simulink model "rw_assembly_step_ramp_test_rpm_commands"  (R2018b)
settings: Solver=FixedStepAuto  StartTime=0.0  StopTime=200  FixedStep=simParams.sample_time_s  RelTol=1e-3
libraries: simulink x1, reaction_wheel_assembly_lib_disc x1
settings Model: Creator=colem  LastModifiedBy=colem

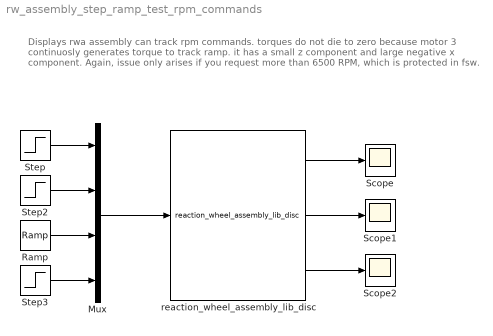
== system rw_assembly_step_ramp_test_rpm_commands ==
  note: Displays rwa assembly can track rpm commands. torques do not die to zero because motor 3 continuosly generates torque to track ramp. it has a small z component and large negative x component. Again, issue only arises if you request more than 6500 RPM, which is protected in fsw.
  Mux : Mux
  Ramp : simulink/Sources/Ramp  slope=6  start=0  InitialOutput=0
  Scope : Scope
  Scope1 : Scope
  Scope2 : Scope
  Step : Step  After=1000  SampleTime=0
  Step2 : Step  After=3000  SampleTime=0
  Step3 : Step  After=-2500  SampleTime=0
  reaction_wheel_assembly_lib_disc : reaction_wheel_assembly_lib_disc/reaction_wheel_assembly_lib_disc  SystemSampleTime=-1
  wires:
  reaction_wheel_assembly_lib_disc/1 -> Scope/1
  reaction_wheel_assembly_lib_disc/2 -> Scope1/1
  reaction_wheel_assembly_lib_disc/3 -> Scope2/1
  Step/1 -> Mux/1
  Step3/1 -> Mux/4
  Step2/1 -> Mux/2
  Mux/1 -> reaction_wheel_assembly_lib_disc/1
  Ramp/1 -> Mux/3
